simulink model "model"  (R2022a)
settings: Solver=FixedStepDiscrete  StartTime=0  StopTime=20  FixedStep=0.01  RelTol=0.00001
model workspace (MAT data in the model file):
  v0 = 0.01
undefined symbols (not defined in the file): alpha, delta, DiscIntNeverNeededParam, Fz, p, s, T, Temp, Tout, vw, ww
libraries: canmsglib x10, MoTeCM1Package x10, simulink x2, slpidlib x1
settings Model: Creator=23326  LastModifiedBy=22793
settings OptimizationCC: LifeSpan=inf
settings DebuggingCC: AlgebraicLoopMsg=none  ArtificialAlgebraicLoopMsg=none  UnconnectedInputMsg=warning  UnconnectedOutputMsg=warning  UnconnectedLineMsg=warning  SFMachineParentedDataDiag=warning  ArithmeticOperatorsInVariantConditions=warning
settings SFSimCC: CustomCodeUndefinedFunction=UseInterfaceOnly
settings CodeAppCC: StateflowObjectComments=on

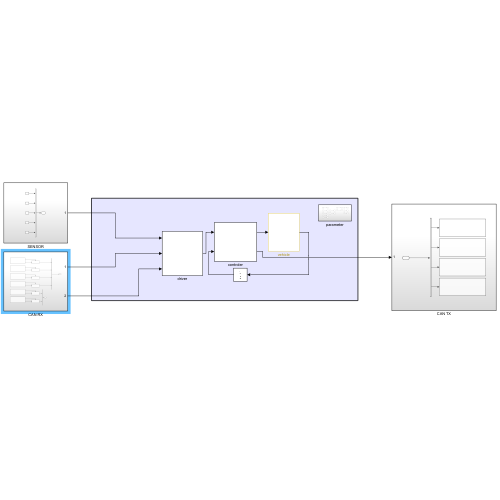
[thumbnail: Simulink's stored preview of the top-level diagram]
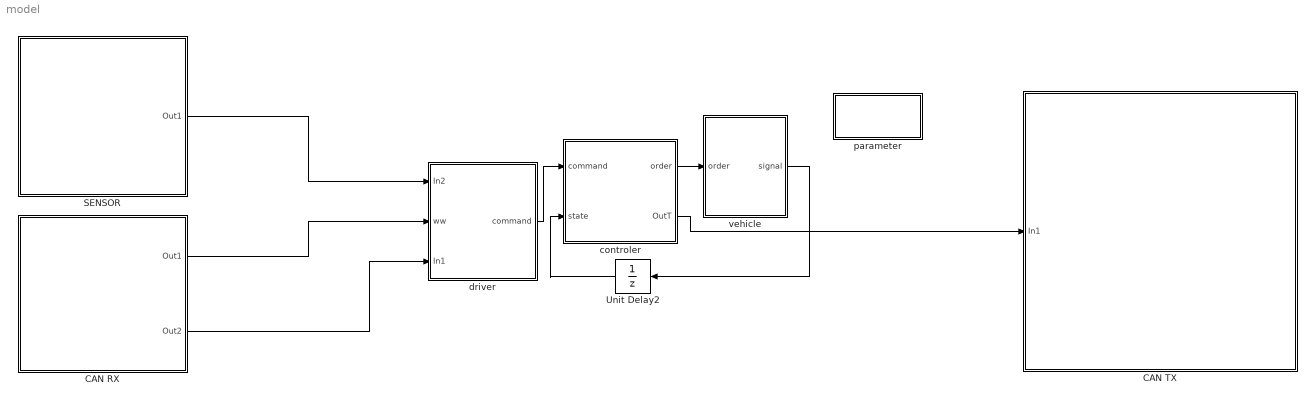
== system model ==
  CAN RX : Subsystem
  CAN TX : Subsystem
  SENSOR : Subsystem
  Unit Delay2 : UnitDelay  SampleTime=-1  HasFrameUpgradeWarning=on
  controler : Subsystem
  driver : Subsystem
  parameter : Subsystem
  vehicle : Subsystem
  wires:
  driver/1(command) -> controler/1(command)
  controler/1(order) -> vehicle/1(order)
  vehicle/1(signal) -> Unit Delay2/1
  Unit Delay2/1 -> controler/2(state)
  controler/2(OutT) -> CAN TX/1(In1)
  SENSOR/1(Out1) -> driver/1(In2)
  CAN RX/1(Out1) -> driver/2(ww)
  CAN RX/2(Out2) -> driver/3(In1)

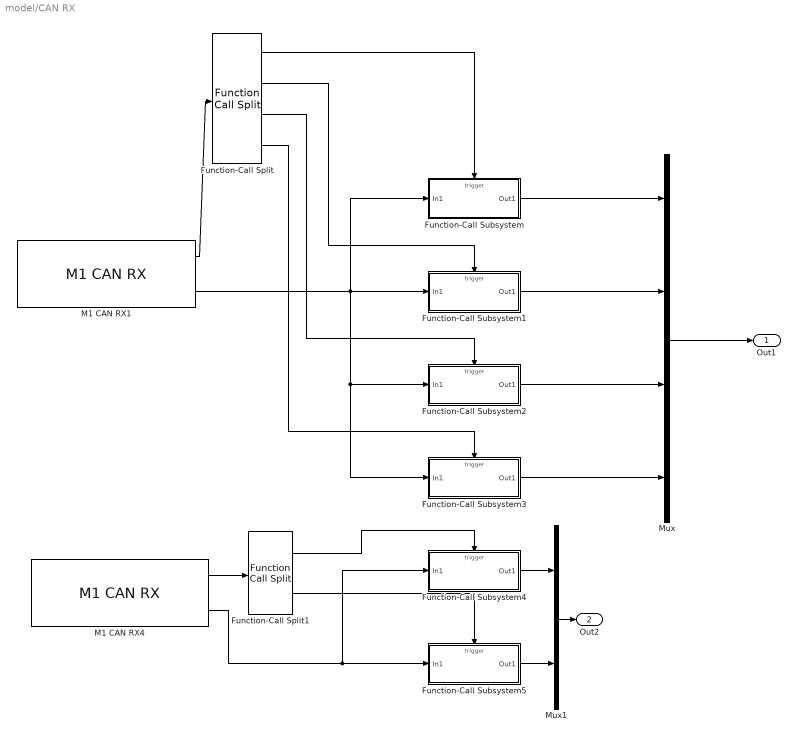
== system model/CAN RX ==
  Function-Call Split : FunctionCallSplit  IconShape=distinctive  NumOutputPorts=4  OutputPortLayout=default
  Function-Call Split1 : FunctionCallSplit  IconShape=distinctive  NumOutputPorts=2  OutputPortLayout=default
  Function-Call Subsystem : Subsystem  TreatAsAtomicUnit=on
  Function-Call Subsystem1 : Subsystem  TreatAsAtomicUnit=on
  Function-Call Subsystem2 : Subsystem  TreatAsAtomicUnit=on
  Function-Call Subsystem3 : Subsystem  TreatAsAtomicUnit=on
  Function-Call Subsystem4 : Subsystem  TreatAsAtomicUnit=on
  Function-Call Subsystem5 : Subsystem  TreatAsAtomicUnit=on
  M1 CAN RX1 : MoTeCM1Package/M1 CAN RX  CANBus=CAN Bus 1  CANFilter=Standard IDs Only  CANIDs=0  SampleTime=-1
      settings: SourceProductName=MoTeC
  M1 CAN RX4 : MoTeCM1Package/M1 CAN RX  CANBus=CAN Bus 1  CANFilter=Standard IDs Only  CANIDs=0  SampleTime=-1
      settings: SourceProductName=MoTeC
  Mux : Mux
  Mux1 : Mux  Inputs=2
  Out1 : Outport
  Out2 : Outport  Port=2
  wires:
  Function-Call Subsystem/1(Out1) -> Mux/1
  Function-Call Subsystem1/1(Out1) -> Mux/2
  Function-Call Subsystem2/1(Out1) -> Mux/3
  Function-Call Subsystem3/1(Out1) -> Mux/4
  Mux/1 -> Out1/1
  Function-Call Subsystem4/1(Out1) -> Mux1/1
  Function-Call Subsystem5/1(Out1) -> Mux1/2
  Mux1/1 -> Out2/1
  Function-Call Split/1 -> Function-Call Subsystem/Trigger
  Function-Call Split/2 -> Function-Call Subsystem1/Trigger
  Function-Call Split/3 -> Function-Call Subsystem2/Trigger
  M1 CAN RX1/2 -> Function-Call Subsystem1/1(In1), Function-Call Subsystem/1(In1), Function-Call Subsystem2/1(In1), Function-Call Subsystem3/1(In1)
  Function-Call Split/4 -> Function-Call Subsystem3/Trigger
  M1 CAN RX4/2 -> Function-Call Subsystem4/1(In1), Function-Call Subsystem5/1(In1)
  Function-Call Split1/2 -> Function-Call Subsystem5/Trigger
  M1 CAN RX1/1 -> Function-Call Split/1
  M1 CAN RX4/1 -> Function-Call Split1/1
  Function-Call Split1/1 -> Function-Call Subsystem4/Trigger

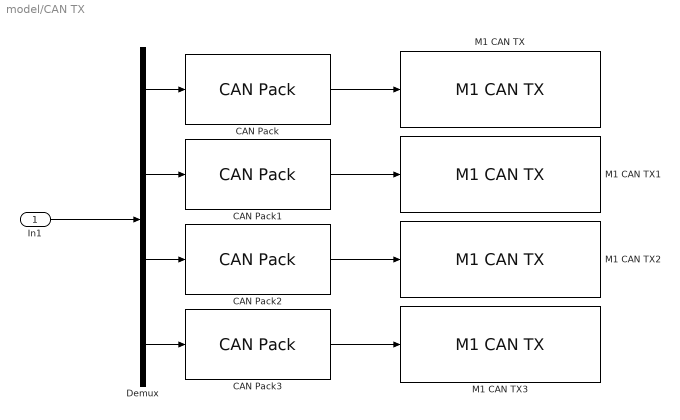
== system model/CAN TX ==
  In1 : Inport
  CAN Pack : canmsglib/CAN Pack  MsgList=(none)  MsgName=CAN Msg  MsgIDType=Standard (11-bit identifier)  MsgIdentifier=0x184  MsgLength=8  Remote=off  ApplyMinMax=off  BusOutput=off  SignalInfo={ 'Signal1', '0', '8', 'LE', 'signed', 'Standard', '0', '1', '32', '-Inf', 'Inf' }
      settings: SourceProductBaseCode=XP,ME,VN  DataFormat=manually specified signals
  CAN Pack1 : canmsglib/CAN Pack  MsgList=(none)  MsgName=CAN Msg  MsgIDType=Standard (11-bit identifier)  MsgIdentifier=0x185  MsgLength=8  Remote=off  ApplyMinMax=off  BusOutput=off  SignalInfo={ 'Signal1', '0', '8', 'LE', 'signed', 'Standard', '0', '1', '32', '-Inf', 'Inf' }
      settings: SourceProductBaseCode=XP,ME,VN  DataFormat=manually specified signals
  CAN Pack2 : canmsglib/CAN Pack  MsgList=(none)  MsgName=CAN Msg  MsgIDType=Standard (11-bit identifier)  MsgIdentifier=0x188  MsgLength=8  Remote=off  ApplyMinMax=off  BusOutput=off  SignalInfo={ 'Signal1', '0', '8', 'LE', 'signed', 'Standard', '0', '1', '32', '-Inf', 'Inf' }
      settings: SourceProductBaseCode=XP,ME,VN  DataFormat=manually specified signals
  CAN Pack3 : canmsglib/CAN Pack  MsgList=(none)  MsgName=CAN Msg  MsgIDType=Standard (11-bit identifier)  MsgIdentifier=0x189  MsgLength=8  Remote=off  ApplyMinMax=off  BusOutput=off  SignalInfo={ 'Signal1', '0', '8', 'LE', 'signed', 'Standard', '0', '1', '32', '-Inf', 'Inf' }
      settings: SourceProductBaseCode=XP,ME,VN  DataFormat=manually specified signals
  Demux : Demux
  M1 CAN TX{,1..3} (4 alike) : MoTeCM1Package/M1 CAN TX  CANBus=CAN Bus 2
      settings: SourceProductName=MoTeC
  wires:
  In1/1 -> Demux/1
  CAN Pack/1 -> M1 CAN TX/1
  Demux/1 -> CAN Pack/1
  Demux/2 -> CAN Pack1/1
  CAN Pack1/1 -> M1 CAN TX1/1
  Demux/3 -> CAN Pack2/1
  CAN Pack2/1 -> M1 CAN TX2/1
  Demux/4 -> CAN Pack3/1
  CAN Pack3/1 -> M1 CAN TX3/1

== system model/SENSOR ==
  Analogue Voltage : MoTeCM1Package/Analogue Voltage  Unit=V  DPS=3  VoltageUpdateRate=10 Hz  SensorUpdateRate=10 Hz  ValType=None  ValMinOn=on  ValMin=0  ValMaxOn=on  ValMax=0  LogRate=Default (Scheduled Rate)  DiagnosticLog=off  DiagnosticLogRate=Default (Log Rate)  SimValue=0  SimStatus=0  SimDiagnostic=0  SimVoltage=0  CRC=1061432025
      settings: SourceProductName=MoTeC
  Analogue Voltage1 : MoTeCM1Package/Analogue Voltage  Unit=V  DPS=3  VoltageUpdateRate=10 Hz  SensorUpdateRate=10 Hz  ValType=None  ValMinOn=on  ValMin=0  ValMaxOn=on  ValMax=0  LogRate=Default (Scheduled Rate)  DiagnosticLog=off  DiagnosticLogRate=Default (Log Rate)  SimValue=0  SimStatus=0  SimDiagnostic=0  SimVoltage=0  CRC=1061432025
      settings: SourceProductName=MoTeC
  Analogue Voltage2 : MoTeCM1Package/Analogue Voltage  Unit=V  DPS=3  VoltageUpdateRate=10 Hz  SensorUpdateRate=10 Hz  ValType=None  ValMinOn=on  ValMin=0  ValMaxOn=on  ValMax=0  LogRate=Default (Scheduled Rate)  DiagnosticLog=off  DiagnosticLogRate=Default (Log Rate)  SimValue=0  SimStatus=0  SimDiagnostic=0  SimVoltage=0  CRC=1061432025
      settings: SourceProductName=MoTeC
  Dual Potentiometer Pedal : MoTeCM1Package/Dual Potentiometer Pedal  Unit=ratio  DPS=3  SensorUpdateRate=50 Hz  ValType=None  ValMinOn=on  ValMin=0  ValMaxOn=on  ValMax=0  LogRate=Default (Scheduled Rate)  DiagnosticLog=off  DiagnosticLogRate=Default (Log Rate)  SimValue=0  SimStatus=0  SimDiagnostic=0  SimMainVoltage=0  SimTrackingVoltage=0  CRC=1697510422
      settings: SourceProductName=MoTeC
  Mux : Mux  Inputs=5
  Out1 : Outport
  wires:
  Analogue Voltage/1 -> Mux/3
  Mux/1 -> Out1/1
  Dual Potentiometer Pedal/1 -> Mux/2, Mux/1
  Analogue Voltage1/1 -> Mux/4
  Analogue Voltage2/1 -> Mux/5

== system model/controler ==
  command : Inport
  state : Inport  Port=2
  Bus Selector : BusSelector  OutputSignals=T
  Constant : Constant  Value=123.9
  Divide : Product  Inputs=*/
  Subsystem : Subsystem
  order : Outport
  OutT : Outport  Port=2
  wires:
  command/1 -> Subsystem/1(Command)
  state/1 -> Subsystem/2(State)
  Subsystem/1(order) -> Bus Selector/1, order/1
  Divide/1 -> OutT/1
  Bus Selector/1 -> Divide/1  "<T>"
  Constant/1 -> Divide/2

== system model/driver ==
  In2 : Inport
  ww : Inport  Port=2
  In1 : Inport  Port=3
  Bus Creator : BusCreator  Inputs=Tout,delta,Temp
  Constant2 : Constant  Value=50
  Demux : Demux  Outputs=5
  Mux : Mux  Inputs=2
  T_control : Subsystem
  command : Outport
  wires:
  Bus Creator/1 -> command/1
  Mux/1 -> Bus Creator/2  "delta"
  Constant2/1 -> Mux/2
  T_control/1(Tout) -> Bus Creator/1  "Tout"
  ww/1 -> T_control/4(ww)
  In1/1 -> Bus Creator/3
  Demux/1 -> T_control/1(Racc)
  Demux/2 -> T_control/2(Lacc)
  Demux/3 -> T_control/3(Brake)
  Demux/4 -> T_control/5(SOC)
  Demux/5 -> Mux/1
  In2/1 -> Demux/1

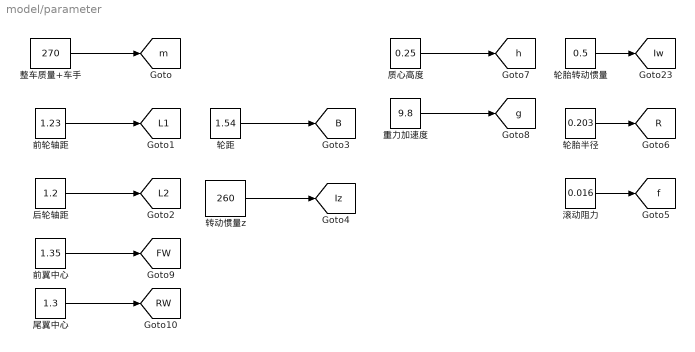
== system model/parameter ==
  前翼中心 : Constant  Value=1.35  OutDataTypeStr=double
  前轮轴距 : Constant  Value=1.23  OutDataTypeStr=double
  后轮轴距 : Constant  Value=1.2  OutDataTypeStr=double
  尾翼中心 : Constant  Value=1.3  OutDataTypeStr=double
  整车质量+车手 : Constant  Value=270  OutDataTypeStr=double
  滚动阻力 : Constant  Value=0.016  OutDataTypeStr=double
  质心高度 : Constant  Value=0.25  OutDataTypeStr=double
  转动惯量z : Constant  Value=260  OutDataTypeStr=double
  轮胎半径 : Constant  Value=0.203  OutDataTypeStr=double
  轮胎转动惯量 : Constant  Value=0.5  OutDataTypeStr=double
  轮距 : Constant  Value=1.54  OutDataTypeStr=double
  重力加速度 : Constant  Value=9.8  OutDataTypeStr=double
  tag scope: B=global, FW=global, Iw=global, Iz=global, L1=global, L2=global, R=global, RW=global, f=global, g=global, h=global, m=global
  wires:
  滚动阻力/1 -> [f]
  轮胎转动惯量/1 -> [Iw]
  整车质量+车手/1 -> [m]
  轮胎半径/1 -> [R]
  后轮轴距/1 -> [L2]
  质心高度/1 -> [h]
  转动惯量z/1 -> [Iz]
  前轮轴距/1 -> [L1]
  轮距/1 -> [B]
  重力加速度/1 -> [g]
  前翼中心/1 -> [FW]
  尾翼中心/1 -> [RW]

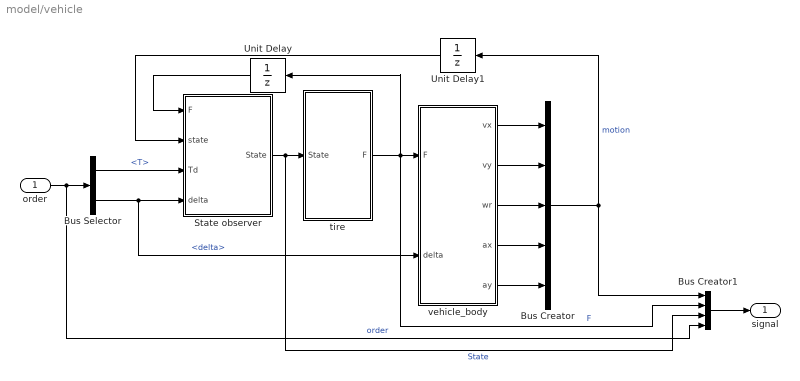
== system model/vehicle ==
  order : Inport
  Bus Creator : BusCreator  Inputs=5
  Bus Creator1 : BusCreator  Inputs=4
  Bus Selector : BusSelector  OutputSignals=T,delta
  State observer : Subsystem
  Unit Delay : UnitDelay  SampleTime=-1  HasFrameUpgradeWarning=on
  Unit Delay1 : UnitDelay  SampleTime=-1  HasFrameUpgradeWarning=on
  tire : Subsystem
  vehicle_body : Subsystem
  signal : Outport
  wires:
  vehicle_body/3(wr) -> Bus Creator/3
  vehicle_body/2(vy) -> Bus Creator/2
  tire/1(F) -> Unit Delay/1, Bus Creator1/2, vehicle_body/1(F)  "F"
  vehicle_body/4(ax) -> Bus Creator/4
  vehicle_body/5(ay) -> Bus Creator/5
  Bus Creator/1 -> Bus Creator1/1, Unit Delay1/1  "motion"
  order/1 -> Bus Creator1/4, Bus Selector/1  "order"
  Bus Selector/1 -> State observer/3(Td)  "<T>"
  Bus Selector/2 -> State observer/4(delta), vehicle_body/2(delta)  "<delta>"
  vehicle_body/1(vx) -> Bus Creator/1
  State observer/1(State) -> Bus Creator1/3, tire/1(State)  "State"
  Bus Creator1/1 -> signal/1
  Unit Delay/1 -> State observer/1(F)
  Unit Delay1/1 -> State observer/2(state)

== system model/CAN RX/Function-Call Subsystem ==
  In1 : Inport
  function : TriggerPort  TriggerType=function-call  VariantControl=(inherit)
  CAN Unpack : canmsglib/CAN Unpack  MsgList=(none)  MsgName=CAN Msg  MsgIDType=Standard (11-bit identifier)  MsgIdentifier=0x283  MsgLength=8  SignalInfo={ 'Signal1', '0', '8', 'LE', 'signed', 'Standard', '0', '1', '16', '-Inf', 'Inf' }  IDPort=off  TimestampPort=off  ErrorPort=off  RemotePort=off  LengthPort=off  StatusPort=off  ApplyMinMax=off
      settings: SourceProductBaseCode=XP,ME,VN
  Out1 : Outport
  wires:
  CAN Unpack/1 -> Out1/1
  In1/1 -> CAN Unpack/1

== system model/CAN RX/Function-Call Subsystem1 ==
  In1 : Inport
  function : TriggerPort  TriggerType=function-call  VariantControl=(inherit)
  CAN Unpack : canmsglib/CAN Unpack  MsgList=(none)  MsgName=CAN Msg  MsgIDType=Standard (11-bit identifier)  MsgIdentifier=0x284  MsgLength=8  SignalInfo={ 'Signal1', '0', '8', 'LE', 'signed', 'Standard', '0', '1', '16', '-Inf', 'Inf' }  IDPort=off  TimestampPort=off  ErrorPort=off  RemotePort=off  LengthPort=off  StatusPort=off  ApplyMinMax=off
      settings: SourceProductBaseCode=XP,ME,VN
  Out1 : Outport
  wires:
  CAN Unpack/1 -> Out1/1
  In1/1 -> CAN Unpack/1

== system model/CAN RX/Function-Call Subsystem2 ==
  In1 : Inport
  function : TriggerPort  TriggerType=function-call  VariantControl=(inherit)
  CAN Unpack : canmsglib/CAN Unpack  MsgList=(none)  MsgName=CAN Msg  MsgIDType=Standard (11-bit identifier)  MsgIdentifier=0x287  MsgLength=8  SignalInfo={ 'Signal1', '0', '8', 'LE', 'signed', 'Standard', '0', '1', '16', '-Inf', 'Inf' }  IDPort=off  TimestampPort=off  ErrorPort=off  RemotePort=off  LengthPort=off  StatusPort=off  ApplyMinMax=off
      settings: SourceProductBaseCode=XP,ME,VN
  Out1 : Outport
  wires:
  In1/1 -> CAN Unpack/1
  CAN Unpack/1 -> Out1/1

== system model/CAN RX/Function-Call Subsystem3 ==
  In1 : Inport
  function : TriggerPort  TriggerType=function-call  VariantControl=(inherit)
  CAN Unpack : canmsglib/CAN Unpack  MsgList=(none)  MsgName=CAN Msg  MsgIDType=Standard (11-bit identifier)  MsgIdentifier=0x288  MsgLength=8  SignalInfo={ 'Signal1', '0', '8', 'LE', 'signed', 'Standard', '0', '1', '16', '-Inf', 'Inf' }  IDPort=off  TimestampPort=off  ErrorPort=off  RemotePort=off  LengthPort=off  StatusPort=off  ApplyMinMax=off
      settings: SourceProductBaseCode=XP,ME,VN
  Out1 : Outport
  wires:
  In1/1 -> CAN Unpack/1
  CAN Unpack/1 -> Out1/1

== system model/CAN RX/Function-Call Subsystem4 ==
  In1 : Inport
  function : TriggerPort  TriggerType=function-call  VariantControl=(inherit)
  CAN Unpack : canmsglib/CAN Unpack  MsgList=(none)  MsgName=CAN Msg  MsgIDType=Standard (11-bit identifier)  MsgIdentifier=0x289  MsgLength=8  SignalInfo={ 'Signal1', '0', '8', 'LE', 'signed', 'Standard', '0', '1', '16', '-Inf', 'Inf' }  IDPort=off  TimestampPort=off  ErrorPort=off  RemotePort=off  LengthPort=off  StatusPort=off  ApplyMinMax=off
      settings: SourceProductBaseCode=XP,ME,VN
  Out1 : Outport
  wires:
  In1/1 -> CAN Unpack/1
  CAN Unpack/1 -> Out1/1

== system model/CAN RX/Function-Call Subsystem5 ==
  In1 : Inport
  function : TriggerPort  TriggerType=function-call  VariantControl=(inherit)
  CAN Unpack : canmsglib/CAN Unpack  MsgList=(none)  MsgName=CAN Msg  MsgIDType=Standard (11-bit identifier)  MsgIdentifier=0x290  MsgLength=8  SignalInfo={ 'Signal1', '0', '8', 'LE', 'signed', 'Standard', '0', '1', '16', '-Inf', 'Inf' }  IDPort=off  TimestampPort=off  ErrorPort=off  RemotePort=off  LengthPort=off  StatusPort=off  ApplyMinMax=off
      settings: SourceProductBaseCode=XP,ME,VN
  Out1 : Outport
  wires:
  In1/1 -> CAN Unpack/1
  CAN Unpack/1 -> Out1/1

== system model/controler/Subsystem ==
  Command : Inport
  State : Inport  Port=2
  Bus Creator : BusCreator  Inputs=delta,T,p
  Bus Selector : BusSelector  OutputSignals=Tout,delta,Temp
  Bus Selector1 : BusSelector  OutputSignals=State.Fz,State.ww,motion.vx,motion.wr
  Demux : Demux  Outputs=2
  MATLAB Function : MATLAB Function  TreatAsAtomicUnit=on
  Mux : Mux  Inputs=2
  Subsystem : Subsystem
  order : Outport
  wires:
  State/1 -> Bus Selector1/1
  Bus Selector1/1 -> Subsystem/2(Fz)  "<Fz>"
  Bus Selector/1 -> Subsystem/1(Req_T)  "<Tout>"
  Command/1 -> Bus Selector/1
  Bus Selector/2 -> Demux/1, Subsystem/4(delta)  "<delta>"
  Subsystem/2(p) -> Bus Creator/3
  Bus Creator/1 -> order/1
  Subsystem/1(T) -> Bus Creator/2  "T"
  Demux/1 -> MATLAB Function/1(u1)
  Demux/2 -> MATLAB Function/2(u2)
  MATLAB Function/1(f) -> Mux/1
  MATLAB Function/2(r) -> Mux/2
  Mux/1 -> Bus Creator/1  "delta"
  Bus Selector/3 -> Subsystem/3(Temp)  "<Temp>"
  Bus Selector1/2 -> Subsystem/5(ww)  "<ww>"
  Bus Selector1/4 -> Subsystem/7(wreal)  "<wr>"
  Bus Selector1/3 -> Subsystem/6(vx)  "<vx>"

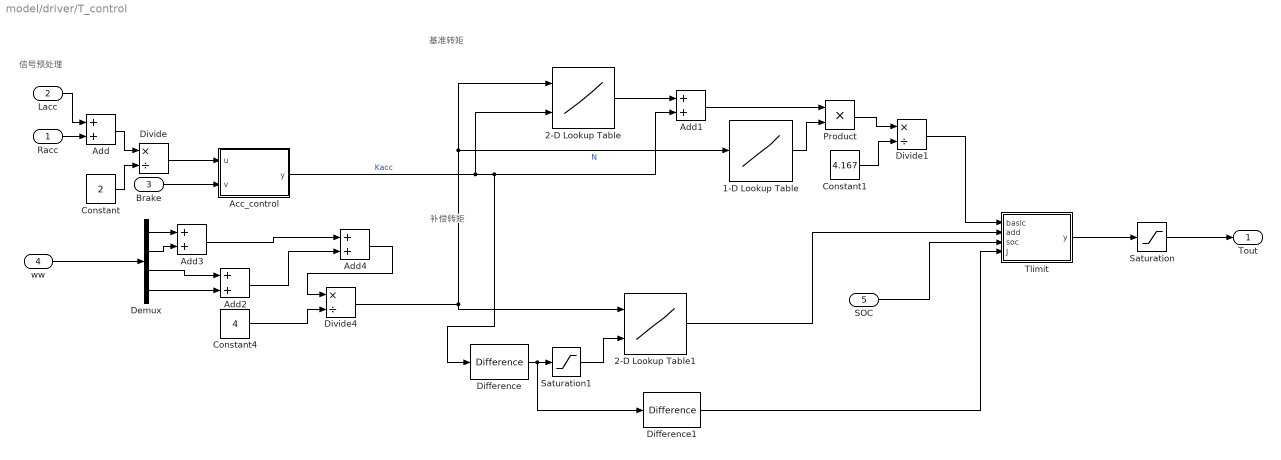
== system model/driver/T_control ==
  note: 补偿转矩
  note: 信号预处理
  note: 基准转矩
  Racc : Inport  OutDataTypeStr=double
  Lacc : Inport  Port=2  OutDataTypeStr=double
  Brake : Inport  Port=3
  ww : Inport  Port=4
  SOC : Inport  Port=5
  1-D Lookup Table : Lookup_n-D  NumberOfTableDimensions=1  BreakpointsForDimension1=[0;1000;2000;3000;4000;5000;6000;7000;8000;9000;10000;11000;12000;13000;14000;15000;16000;17000;18000;19000]  Table=[21;21;21;21;21;21;21;21;21;21;21;21;21;21;20;18;15;13;9.8;0]  InternalRulePriority=Speed  RndMeth=Simplest
  2-D Lookup Table : Lookup_n-D  BreakpointsForDimension1=[0 1000 2000 3000 4000 5000 6000 7000 8000 9000 10000 12000 14000]  BreakpointsForDimension2=[0 5 10 20 30 40 50 60 70 80 90 95 100]  BreakpointsForDimension1FirstPoint=0  BreakpointsForDimension2FirstPoint=0  BreakpointsForDimension1Spacing=1000  BreakpointsForDimension2Spacing=10  Table=[0.315789474 0.653846154 0.703703704 0.80952381 1.052631579 1.194444444 1.302083333 1.507246377 1.564102564 1.507246377 1.564102564 1.527777778 1.564102564;0.342857143 0.666666667 0.666666667 0.768707483 0.930232558 1.068181818 1.088888889 1.419354839 1.419354839 1.419354839 1.419354839 1.419354839 1.507246377;0.315789474 0.513888889 0.533333333 0.62601626 0.583333333 0.422222222 0.627118644 0.871794872 1.052631579 1.147058824 1.225 1.236842105 1.302083333;0.150537634 0.333333333 0.333333333 0.333333333 0.263565891 0.031446541 0.333333333 0.698113208 0.930232558 1.023809524 1.088888889 1.088888889 1.216216216;0.137254902 0.257575758 0.173333333 0.141843972 -0.083333333 -0.31372549 -0.133333333 0.122807018 0.346666667 0.468085106 0.589285714 0.847826087 1.138888889;0.150537634 0.263565891 0.141843972 1.34572e-17 -0.210884354 -0.635220126 -0.542372881 -0.303030303 6.72862e-17 0.237288136 0.58490566 0.837037037 1.121212121;0.137254902 0.12962963 5.28678e-17 -0.141843972 -0.310606061 -0.777777778 -0.724637681 -0.549019608 -0.217391304 0.237288136 0.589285714 0.847826087 1.138888889;1.37065e-17 -0.08045977 -0.212121212 -0.333333333 -0.403100775 -0.635220126 -0.866666667 -0.974358974 -0.290598291 0.237288136 0.58490566 0.837037037 1;1.23358e-17 -0.077777778 -0.194444444 -0.212121212 -0.280701754 -0.511111111 -0.69005848 -0.549019608 -0.217391304 0.192982456 0.4375 0.692982456 0.861111111;1.37065e-17 -0.08045977 -0.212121212 -0.333333333 -0.333333333 -0.333333333 -0.542372881 -0.303030303 -0.06918239 1.45127e-17 0.205128205 0.47311828 0.666666667;-0.194444444 -0.205882353 -0.194444444 -0.333333333 -0.472222222 -0.454545455 -0.385964912 -0.078431373 0.143939394 0.205128205 0.238095238 0.37037037 0.472222222;-0.333333333 -0.333333333 -0.333333333 -0.333333333 -0.454545455 -0.358974359 -0.2 0.333333333 0.333333333 0.333333333 0.333333333 0.333333333 0.333333333;-0.472222222 -0.460784314 -0.472222222 -0.454545455 -0.472222222 -0.358974359 -0.058333333 0.212121212 0.194444444 0.212121212 0.194444444 0.205882353 0.194444444]  InternalRulePriority=Speed  RndMeth=Simplest
      settings: InputPortMap=u0,u1
  2-D Lookup Table1 : Lookup_n-D  BreakpointsForDimension1=[0;1000;2000;3000;4000;5000;6000;7000;8000;9000;10000;11000;12000;13000;14000]  BreakpointsForDimension2=[-50;-25;0;25;50]  Table=[0 0 0 4 5;0 0 0 4 5;0 0 0 4 5;0 0 0 4 5;-3 -2 0 4 5;-3 -2 0 3 5;-3 -2 0 3 4;-3 -2 0 3 4;-4 -3 0 2 3;-4 -3 0 2 3;-5 -3 0 1 2;-5 -4 0 1 2;-5 -4 0 0 0;-5 -4 0 0 0;-5 -4 0 0 0]  InternalRulePriority=Speed  RndMeth=Simplest
      settings: InputPortMap=u0,u1
  Acc_control : MATLAB Function  TreatAsAtomicUnit=on
  Add{,1..4} (5 alike) : Sum
  Constant : Constant  Value=2  OutDataTypeStr=uint8
  Constant1 : Constant  Value=4.167
  Constant4 : Constant  Value=4
  Demux : Demux
  Difference : simulink/Discrete/Difference  ICPrevInput=0.0  OutMin=[]  OutMax=[]  OutDataType=fixdt(1, 16)  OutScaling=2^-10  DoSatur=off
  Difference1 : simulink/Discrete/Difference  ICPrevInput=0.0  OutMin=[]  OutMax=[]  OutDataType=fixdt(1, 16)  OutScaling=2^-10  DoSatur=off
  Divide : Product  Inputs=*/
  Divide1 : Product  Inputs=*/
  Divide4 : Product  Inputs=*/
  Product : Product
  Saturation : Saturate  UpperLimit=495  LowerLimit=0
  Saturation1 : Saturate  UpperLimit=50  LowerLimit=-50
  Tlimit : MATLAB Function  TreatAsAtomicUnit=on
  Tout : Outport
  wires:
  Lacc/1 -> Add/1
  Racc/1 -> Add/2
  Add/1 -> Divide/1
  Constant/1 -> Divide/2
  Brake/1 -> Acc_control/2(v)
  Divide/1 -> Acc_control/1(u)
  SOC/1 -> Tlimit/3(soc)
  Difference/1 -> Difference1/1, Saturation1/1
  Difference1/1 -> Tlimit/4(J)
  1-D Lookup Table/1 -> Product/2
  2-D Lookup Table/1 -> Add1/1
  Demux/3 -> Add2/1
  Demux/4 -> Add2/2
  Constant4/1 -> Divide4/2
  Divide4/1 -> 2-D Lookup Table/1, 1-D Lookup Table/1, 2-D Lookup Table1/1  "N"
  Acc_control/1(y) -> 2-D Lookup Table/2, Difference/1, Add1/2  "Kacc"
  Demux/1 -> Add3/1
  Demux/2 -> Add3/2
  Add3/1 -> Add4/1
  Add2/1 -> Add4/2
  Add4/1 -> Divide4/1
  Saturation/1 -> Tout/1
  Tlimit/1(y) -> Saturation/1
  Saturation1/1 -> 2-D Lookup Table1/2
  Add1/1 -> Product/1
  Product/1 -> Divide1/1
  Constant1/1 -> Divide1/2
  Divide1/1 -> Tlimit/1(basic)
  ww/1 -> Demux/1
  2-D Lookup Table1/1 -> Tlimit/2(add)

== system model/vehicle/State observer ==
  F : Inport
  state : Inport  Port=2
  Td : Inport  Port=3
  delta : Inport  Port=4
  Bus Creator : BusCreator  Inputs=alpha,s,Fz,ww,vw
  Fz : Subsystem
  alpha&vw : Subsystem
  lamda : Subsystem
  wheel : Subsystem
  State : Outport
  wires:
  alpha&vw/1(alpha) -> Bus Creator/1  "alpha"
  Fz/1(Fz) -> wheel/3(Fz), Bus Creator/3  "Fz"
  alpha&vw/2(vw) -> Bus Creator/5, lamda/1(vw)  "vw"
  wheel/1(ww) -> lamda/2(ww), Bus Creator/4  "ww"
  lamda/1(s) -> Bus Creator/2  "s"
  state/1 -> alpha&vw/2(state), Fz/1(state)
  Td/1 -> wheel/1(Td)  "Td"
  Bus Creator/1 -> State/1
  F/1 -> wheel/2(F)
  delta/1 -> alpha&vw/1(delta)

== system model/vehicle/tire ==
  State : Inport
  Bus Creator : BusCreator  Inputs=8
  Bus Selector : BusSelector  OutputSignals=alpha,s,Fz
  MATLAB Function3 : MATLAB Function  TreatAsAtomicUnit=on
  F : Outport
  wires:
  MATLAB Function3/1(Fx1) -> Bus Creator/1
  MATLAB Function3/4(Fx4) -> Bus Creator/4
  MATLAB Function3/3(Fx3) -> Bus Creator/3
  MATLAB Function3/2(Fx2) -> Bus Creator/2
  MATLAB Function3/5(Fy1) -> Bus Creator/5
  MATLAB Function3/6(Fy2) -> Bus Creator/6
  MATLAB Function3/7(Fy3) -> Bus Creator/7
  MATLAB Function3/8(Fy4) -> Bus Creator/8
  State/1 -> Bus Selector/1
  Bus Selector/1 -> MATLAB Function3/1(alpha)  "<alpha>"
  Bus Selector/2 -> MATLAB Function3/2(s)  "<s>"
  Bus Selector/3 -> MATLAB Function3/3(Fz)  "<Fz>"
  Bus Creator/1 -> F/1

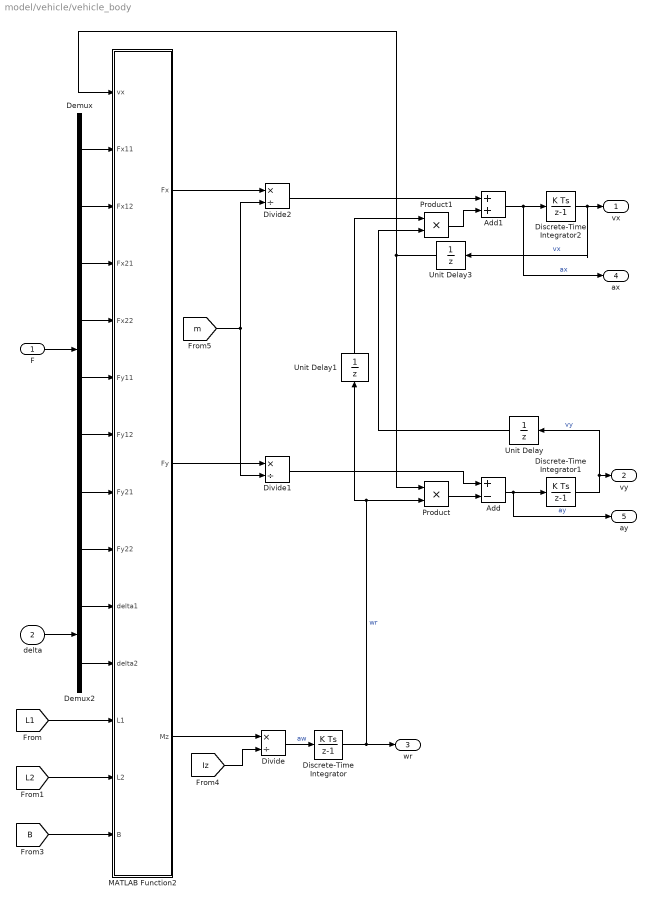
== system model/vehicle/vehicle_body ==
  F : Inport
  delta : Inport  Port=2
  Add : Sum  Inputs=+-
  Add1 : Sum
  Demux : Demux  Outputs=8
  Demux2 : Demux  Outputs=2
  Discrete-Time Integrator : DiscreteIntegrator  SampleTime=-1  ICPrevOutput=DiscIntNeverNeededParam  ICPrevScaledInput=DiscIntNeverNeededParam
  Discrete-Time Integrator1 : DiscreteIntegrator  SampleTime=-1  ICPrevOutput=DiscIntNeverNeededParam  ICPrevScaledInput=DiscIntNeverNeededParam
  Discrete-Time Integrator2 : DiscreteIntegrator  SampleTime=-1  ICPrevOutput=DiscIntNeverNeededParam  ICPrevScaledInput=DiscIntNeverNeededParam
  Divide : Product  Inputs=*/
  Divide1 : Product  Inputs=*/
  Divide2 : Product  Inputs=*/
  MATLAB Function2 : MATLAB Function  TreatAsAtomicUnit=on
  Product : Product
  Product1 : Product
  Unit Delay : UnitDelay  SampleTime=-1  HasFrameUpgradeWarning=on
  Unit Delay1 : UnitDelay  SampleTime=-1  HasFrameUpgradeWarning=on
  Unit Delay3 : UnitDelay  SampleTime=-1  HasFrameUpgradeWarning=on
  vx : Outport
  vy : Outport  Port=2
  wr : Outport  Port=3
  ax : Outport  Port=4
  ay : Outport  Port=5
  wires:
  Discrete-Time Integrator1/1 -> Unit Delay/1, vy/1  "vy"
  Discrete-Time Integrator/1 -> Product/2, Unit Delay1/1, wr/1  "wr"
  Divide/1 -> Discrete-Time Integrator/1  "aw"
  Discrete-Time Integrator2/1 -> vx/1, Unit Delay3/1  "vx"
  Demux2/2 -> MATLAB Function2/11(delta2)
  MATLAB Function2/3(Mz) -> Divide/1
  Add/1 -> Discrete-Time Integrator1/1, ay/1  "ay"
  Divide2/1 -> Add1/1
  Add1/1 -> Discrete-Time Integrator2/1, ax/1  "ax"
  MATLAB Function2/1(Fx) -> Divide2/1
  Divide1/1 -> Add/1
  Product1/1 -> Add1/2
  MATLAB Function2/2(Fy) -> Divide1/1
  Product/1 -> Add/2
  delta/1 -> Demux2/1
  F/1 -> Demux/1
  Demux2/1 -> MATLAB Function2/10(delta1)
  [L1] -> MATLAB Function2/12(L1)
  [L2] -> MATLAB Function2/13(L2)
  [B] -> MATLAB Function2/14(B)
  [Iz] -> Divide/2
  [m] -> Divide2/2, Divide1/2
  Demux/8 -> MATLAB Function2/9(Fy22)
  Demux/7 -> MATLAB Function2/8(Fy21)
  Demux/6 -> MATLAB Function2/7(Fy12)
  Demux/5 -> MATLAB Function2/6(Fy11)
  Demux/4 -> MATLAB Function2/5(Fx22)
  Demux/3 -> MATLAB Function2/4(Fx21)
  Demux/2 -> MATLAB Function2/3(Fx12)
  Demux/1 -> MATLAB Function2/2(Fx11)
  Unit Delay/1 -> Product1/2
  Unit Delay1/1 -> Product1/1
  Unit Delay3/1 -> MATLAB Function2/1(vx), Product/1

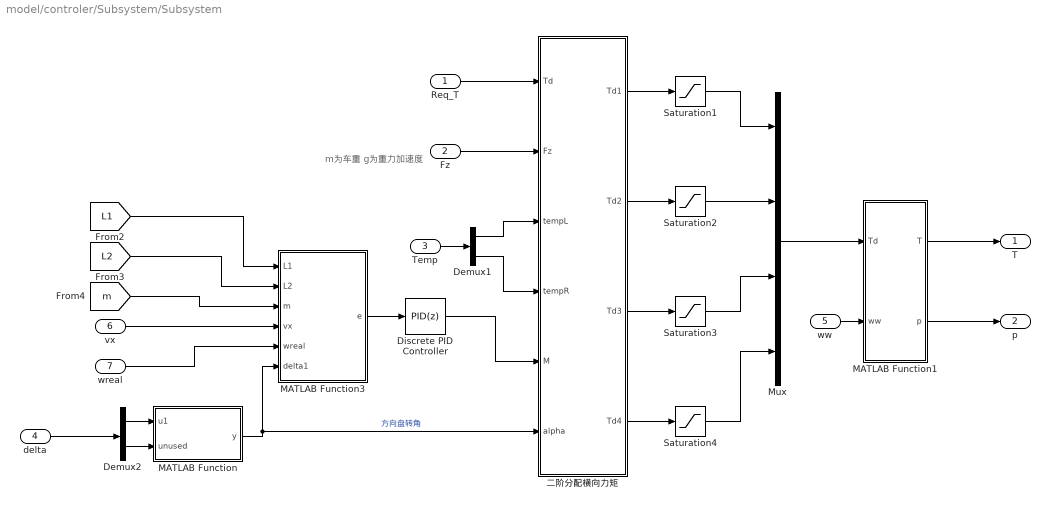
== system model/controler/Subsystem/Subsystem ==
  note: m为车重
      | g为重力加速度
  Req_T : Inport
  Fz : Inport  Port=2
  Temp : Inport  Port=3
  delta : Inport  Port=4
  ww : Inport  Port=5
  vx : Inport  Port=6
  wreal : Inport  Port=7
  Demux1 : Demux  Outputs=2
  Demux2 : Demux  Outputs=2
  Discrete PID Controller : slpidlib/PID Controller  Controller=PID  Form=Parallel  TimeDomain=Discrete-time  UseExternalTs=off  SampleTime=-1  IntegratorMethod=Forward Euler  FilterMethod=Forward Euler  ControllerParametersSource=internal  P=20  I=5  UseKiTs=off  D=2  N=20  UseFilter=on  TunerSelectOption=Frequency Response Based  InitialConditionSource=internal  InitialConditionForIntegrator=0  InitialConditionForFilter=0  DifferentiatorICPrevScaledInput=0  ExternalReset=none  TrackingMode=off  Kt=1  LimitOutput=off  SatLimitsSource=internal  UpperSaturationLimit=inf  LowerSaturationLimit=-inf  LinearizeAsGain=off  AntiWindupMode=none  Kb=1  POutMin=[]  POutMax=[]  IOutMin=[]  IOutMax=[]  DOutMin=[]  DOutMax=[]  NOutMin=[]  NOutMax=[]  SumOutMin=[]  SumOutMax=[]  SaturationOutMin=[]  SaturationOutMax=[]  PParamMin=[]  PParamMax=[]  IParamMin=[]  IParamMax=[]  DParamMin=[]  DParamMax=[]  NParamMin=[]  NParamMax=[]  KbParamMin=[]  KbParamMax=[]  KtParamMin=[]  KtParamMax=[]  KbOutMin=[]  KbOutMax=[]  KtOutMin=[]  KtOutMax=[]  IntegratorOutMin=[]  IntegratorOutMax=[]  FilterOutMin=[]  FilterOutMax=[]  SumI1OutMin=[]  SumI1OutMax=[]  SumI2OutMin=[]  SumI2OutMax=[]  SumI3OutMin=[]  SumI3OutMax=[]  SumI4OutMin=[]  SumI4OutMax=[]  SumDOutMin=[]  SumDOutMax=[]  DifferentiatorOutMin=[]  DifferentiatorOutMax=[]  FilterDiffOutCoefMin=[]  FilterDiffOutCoefMax=[]  ReciprocalOutMin=[]  ReciprocalOutMax=[]  SumDenOutMin=[]  SumDenOutMax=[]  SumNumOutMin=[]  SumNumOutMax=[]  DivideOutMin=[]  DivideOutMax=[]  UdiffTsProdOutMin=[]  UdiffTsProdOutMax=[]  NTsProdOutMin=[]  NTsProdOutMax=[]  UintegralTsProdOutMin=[]  UintegralTsProdOutMax=[]  UngainTsProdOutMin=[]  UngainTsProdOutMax=[]  ClampingZeroOutDataTypeStr=Inherit: Inherit via back propagation  ClampingZeroOutMin=[]  ClampingZeroOutMax=[]  FilterDenConstantOutDataTypeStr=Inherit: Inherit via back propagation  FilterDenConstantOutMin=[]  FilterDenConstantOutMax=[]  PCopyOutDataTypeStr=Inherit: Inherit via back propagation  PCopyOutMin=[]  PCopyOutMax=[]  NCopyOutDataTypeStr=Inherit: Inherit via back propagation  NCopyOutMin=[]  NCopyOutMax=[]  IntegratorContinuousStateAttributes=''  IntegratorStateMustResolveToSignalObject=off  IntegratorRTWStateStorageClass=Auto  FilterContinuousStateAttributes=''  FilterStateMustResolveToSignalObject=off  FilterRTWStateStorageClass=Auto  ParallelPVariant=InternalParameters  IdealPVariant=Disabled  IVariant=InternalParameters  DVariant=InternalParameters  IntegratorVariant=Discrete  SatVariant=Disabled  AWVariant=Passthrough  PCopyVariant=Disabled  TRVariant=Disabled  FdbkBlocksVariant=Forward  IdealPFdbkVariant=Disabled  SatFdbkVariant=Disabled  DerivativeFilterVariant=ForwardEulerFilter  NVariant=InternalParameters  NCopyVariant=Disabled  FilterICVariant=InternalICsFilter  IntegratorICVariant=InternalICs  ExternalResetVariant=Disabled  TRSumVariant=Passthrough  SumFdbkVariant=Disabled  SumVariant=Sum_PID  TsampFilterVariant=InternalTs  TsampNgainVariant=Passthrough  TsampIntegralVariant=Passthrough  ExternalSaturationOutDataTypeStr=Inherit: Same as second input  aMode=0
  MATLAB Function : MATLAB Function  TreatAsAtomicUnit=on
  MATLAB Function1 : MATLAB Function  TreatAsAtomicUnit=on
  MATLAB Function3 : MATLAB Function  TreatAsAtomicUnit=on
  Mux : Mux
  Saturation{1..4} (4 alike) : Saturate  UpperLimit=123.9  LowerLimit=0
  二阶分配横向力矩 : MATLAB Function  TreatAsAtomicUnit=on
  T : Outport
  p : Outport  Port=2
  wires:
  Fz/1 -> 二阶分配横向力矩/2(Fz)
  Demux1/1 -> 二阶分配横向力矩/3(tempL)
  Demux2/1 -> MATLAB Function/1(u1)
  Req_T/1 -> 二阶分配横向力矩/1(Td)
  Demux1/2 -> 二阶分配横向力矩/4(tempR)
  delta/1 -> Demux2/1
  Temp/1 -> Demux1/1
  Demux2/2 -> MATLAB Function/2(unused)
  二阶分配横向力矩/1(Td1) -> Saturation1/1
  二阶分配横向力矩/2(Td2) -> Saturation2/1
  二阶分配横向力矩/3(Td3) -> Saturation3/1
  二阶分配横向力矩/4(Td4) -> Saturation4/1
  ww/1 -> MATLAB Function1/2(ww)
  Saturation1/1 -> Mux/1
  Saturation2/1 -> Mux/2
  Saturation3/1 -> Mux/3
  Saturation4/1 -> Mux/4
  Mux/1 -> MATLAB Function1/1(Td)
  MATLAB Function1/2(p) -> p/1
  MATLAB Function1/1(T) -> T/1
  vx/1 -> MATLAB Function3/4(vx)
  wreal/1 -> MATLAB Function3/5(wreal)
  [m] -> MATLAB Function3/3(m)
  [L2] -> MATLAB Function3/2(L2)
  [L1] -> MATLAB Function3/1(L1)
  MATLAB Function/1(y) -> 二阶分配横向力矩/6(alpha), MATLAB Function3/6(delta1)  "方向盘转角"
  MATLAB Function3/1(e) -> Discrete PID Controller/1
  Discrete PID Controller/1 -> 二阶分配横向力矩/5(M)

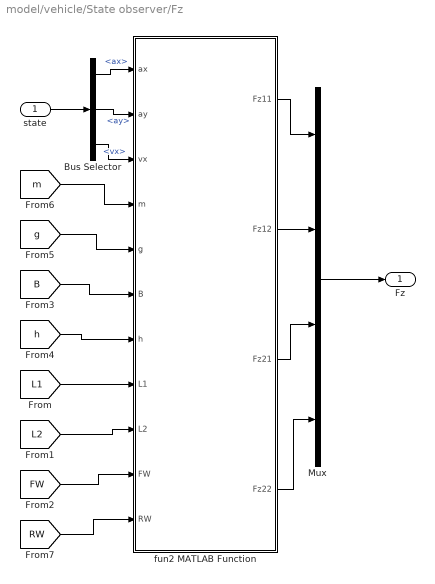
== system model/vehicle/State observer/Fz ==
  state : Inport
  Bus Selector : BusSelector  OutputSignals=ax,ay,vx
  Mux : Mux
  fun2 MATLAB Function : MATLAB Function  TreatAsAtomicUnit=on
  Fz : Outport
  wires:
  [L2] -> fun2 MATLAB Function/9(L2)
  [L1] -> fun2 MATLAB Function/8(L1)
  [h] -> fun2 MATLAB Function/7(h)
  [g] -> fun2 MATLAB Function/5(g)
  [m] -> fun2 MATLAB Function/4(m)
  Mux/1 -> Fz/1
  fun2 MATLAB Function/1(Fz11) -> Mux/1
  fun2 MATLAB Function/2(Fz12) -> Mux/2
  fun2 MATLAB Function/3(Fz21) -> Mux/3
  fun2 MATLAB Function/4(Fz22) -> Mux/4
  [B] -> fun2 MATLAB Function/6(B)
  state/1 -> Bus Selector/1
  Bus Selector/1 -> fun2 MATLAB Function/1(ax)  "<ax>"
  Bus Selector/2 -> fun2 MATLAB Function/2(ay)  "<ay>"
  Bus Selector/3 -> fun2 MATLAB Function/3(vx)  "<vx>"
  [FW] -> fun2 MATLAB Function/10(FW)
  [RW] -> fun2 MATLAB Function/11(RW)

== system model/vehicle/State observer/alpha&vw ==
  delta : Inport
  state : Inport  Port=2
  Bus Selector : BusSelector  OutputSignals=vx,vy,wr
  cepianjiao : Subsystem
  lunsu : Subsystem
  alpha : Outport
  vw : Outport  Port=2
  wires:
  lunsu/1(vw) -> vw/1
  Bus Selector/2 -> lunsu/3(vy), cepianjiao/3(vy)  "<vy>"
  cepianjiao/1(alpha) -> alpha/1
  delta/1 -> lunsu/1(delta), cepianjiao/1(delta)
  Bus Selector/1 -> cepianjiao/2(vx), lunsu/2(vx)  "<vx>"
  state/1 -> Bus Selector/1
  Bus Selector/3 -> lunsu/4(wr), cepianjiao/4(wr)  "<wr>"

== system model/vehicle/State observer/lamda ==
  vw : Inport
  ww : Inport  Port=2
  MATLAB Function2 : MATLAB Function  TreatAsAtomicUnit=on
  Mux : Mux
  s : Outport
  wires:
  [R] -> MATLAB Function2/3(R)
  vw/1 -> MATLAB Function2/1(vw)
  ww/1 -> MATLAB Function2/2(ww)
  MATLAB Function2/1(s1) -> Mux/1
  MATLAB Function2/4(s4) -> Mux/4
  MATLAB Function2/2(s2) -> Mux/2
  MATLAB Function2/3(s3) -> Mux/3
  Mux/1 -> s/1

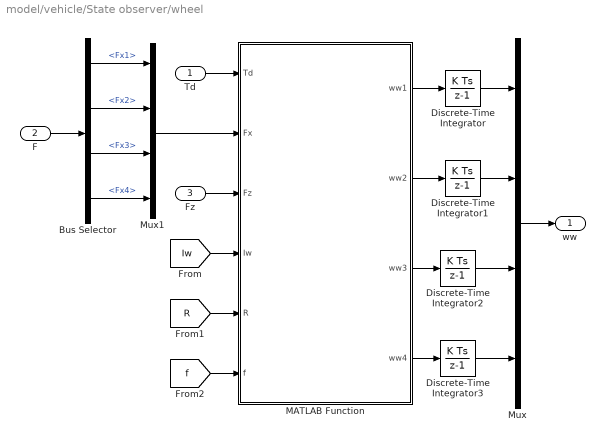
== system model/vehicle/State observer/wheel ==
  Td : Inport
  F : Inport  Port=2
  Fz : Inport  Port=3
  Bus Selector : BusSelector  OutputSignals=Fx1,Fx2,Fx3,Fx4
  Discrete-Time Integrator{,1..3} (4 alike) : DiscreteIntegrator  SampleTime=-1  ICPrevOutput=DiscIntNeverNeededParam  ICPrevScaledInput=DiscIntNeverNeededParam
  MATLAB Function : MATLAB Function  TreatAsAtomicUnit=on
  Mux : Mux
  Mux1 : Mux
  ww : Outport
  wires:
  MATLAB Function/1(ww1) -> Discrete-Time Integrator/1
  Discrete-Time Integrator/1 -> Mux/1
  Td/1 -> MATLAB Function/1(Td)
  Fz/1 -> MATLAB Function/3(Fz)
  Discrete-Time Integrator1/1 -> Mux/2
  Discrete-Time Integrator2/1 -> Mux/3
  Discrete-Time Integrator3/1 -> Mux/4
  [Iw] -> MATLAB Function/4(Iw)
  [R] -> MATLAB Function/5(R)
  [f] -> MATLAB Function/6(f)
  Mux/1 -> ww/1
  MATLAB Function/2(ww2) -> Discrete-Time Integrator1/1
  MATLAB Function/3(ww3) -> Discrete-Time Integrator2/1
  MATLAB Function/4(ww4) -> Discrete-Time Integrator3/1
  F/1 -> Bus Selector/1
  Bus Selector/1 -> Mux1/1  "<Fx1>"
  Bus Selector/2 -> Mux1/2  "<Fx2>"
  Bus Selector/3 -> Mux1/3  "<Fx3>"
  Bus Selector/4 -> Mux1/4  "<Fx4>"
  Mux1/1 -> MATLAB Function/2(Fx)

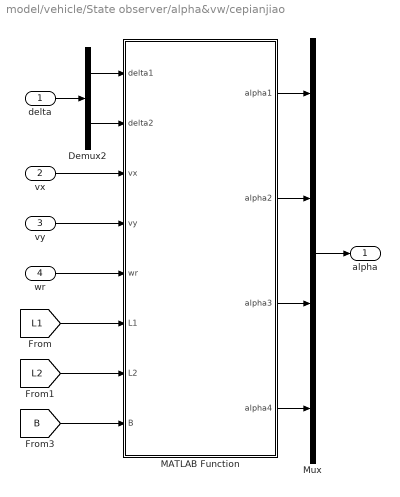
== system model/vehicle/State observer/alpha&vw/cepianjiao ==
  delta : Inport
  vx : Inport  Port=2
  vy : Inport  Port=3
  wr : Inport  Port=4
  Demux2 : Demux  Outputs=2
  MATLAB Function : MATLAB Function  TreatAsAtomicUnit=on
  Mux : Mux
  alpha : Outport
  wires:
  vy/1 -> MATLAB Function/4(vy)
  vx/1 -> MATLAB Function/3(vx)
  wr/1 -> MATLAB Function/5(wr)
  Demux2/1 -> MATLAB Function/1(delta1)
  delta/1 -> Demux2/1
  Demux2/2 -> MATLAB Function/2(delta2)
  [L1] -> MATLAB Function/6(L1)
  [L2] -> MATLAB Function/7(L2)
  [B] -> MATLAB Function/8(B)
  Mux/1 -> alpha/1
  MATLAB Function/1(alpha1) -> Mux/1
  MATLAB Function/2(alpha2) -> Mux/2
  MATLAB Function/3(alpha3) -> Mux/3
  MATLAB Function/4(alpha4) -> Mux/4

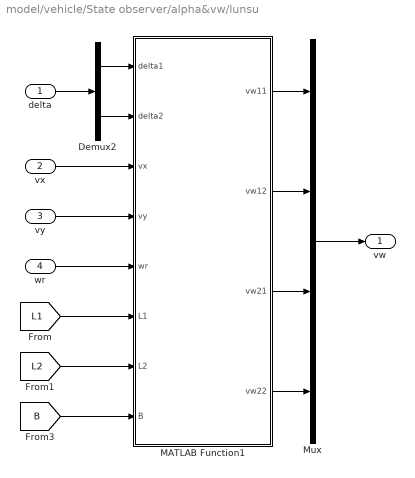
== system model/vehicle/State observer/alpha&vw/lunsu ==
  delta : Inport
  vx : Inport  Port=2
  vy : Inport  Port=3
  wr : Inport  Port=4
  Demux2 : Demux  Outputs=2
  MATLAB Function1 : MATLAB Function  TreatAsAtomicUnit=on
  Mux : Mux
  vw : Outport
  wires:
  Demux2/1 -> MATLAB Function1/1(delta1)
  vy/1 -> MATLAB Function1/4(vy)
  vx/1 -> MATLAB Function1/3(vx)
  [B] -> MATLAB Function1/8(B)
  [L2] -> MATLAB Function1/7(L2)
  Demux2/2 -> MATLAB Function1/2(delta2)
  wr/1 -> MATLAB Function1/5(wr)
  delta/1 -> Demux2/1
  [L1] -> MATLAB Function1/6(L1)
  Mux/1 -> vw/1
  MATLAB Function1/1(vw11) -> Mux/1
  MATLAB Function1/2(vw12) -> Mux/2
  MATLAB Function1/3(vw21) -> Mux/3
  MATLAB Function1/4(vw22) -> Mux/4

== matlab function model/vehicle/State observer/lamda/MATLAB Function2 ==
  data: vw input size=4; ww input size=4; s1 output; R input; s2 output; s3 output; s4 output
function [s1,s2,s3,s4] = fcn(vw,ww,R) 

s1 = (ww(1)*R-vw(1))/max(vw(1),ww(1)*R)*100;
s2 = (ww(2)*R-vw(2))/max(vw(2),ww(2)*R)*100;
s3 = (ww(3)*R-vw(3))/max(vw(3),ww(3)*R)*100;
s4 = (ww(4)*R-vw(4))/max(vw(4),ww(4)*R)*100;

== matlab function model/vehicle/tire/MATLAB Function3 ==
  data: alpha input size=4; s input size=4; Fz input size=4; Fx1 output; Fx2 output; Fx3 output; Fx4 output; Fy1 output; Fy2 output; Fy3 output; Fy4 output
function [Fx1,Fx2,Fx3,Fx4,Fy1,Fy2,Fy3,Fy4]= fcn(alpha,s,Fz)
alpha=alpha*180/pi;
miu=1;
%%纵向力与侧向力计算
% Cx=20000;
% Cy=30000;
% l11=miu*Fz(1)*(1+s(1))/2/sqrt((Cx*s(1))^2+(Cy*tan(alpha(1)))^2);
% l12=miu*Fz(2)*(1+s(2))/2/sqrt((Cx*s(2))^2+(Cy*tan(alpha(2)))^2);
% l21=miu*Fz(3)*(1+s(3))/2/sqrt((Cx*s(3))^2+(Cy*tan(alpha(3)))^2);
% l22=miu*Fz(4)*(1+s(4))/2/sqrt((Cx*s(4))^2+(Cy*tan(alpha(4)))^2);
% %状态函数判断
% if l11<1
%     f11=l11*(2-l11);
% else
%     f11=1;
% end
% if l12<1
%     f12=l12*(2-l12);
% else
%     f12=1;
% end
% if l21<1
%     f21=l21*(2-l21);
% else
%     f21=1;
% end
% if l22<1
%     f22=l22*(2-l22);
% else
%     f22=1;
% end
% %纵向力与横向力计算
% Fx1=Cx*s(1)*f11/(1+s(1));
% Fy1=Cy*tan(alpha(1))*f11/(1+s(1));
% Fx2=Cx*s(2)*f12/(1+s(2));
% Fy2=Cy*tan(alpha(2))*f12/(1+s(2));
% Fx3=Cx*s(3)*f21/(1+s(3));
% Fy3=Cy*tan(alpha(3))*f21/(1+s(3));
% Fx4=Cx*s(4)*f22/(1+s(4));
% Fy4=Cy*tan(alpha(4))*f22/(1+s(4));
Fz=Fz/1000;

%% 11
a1=-21.3;a2=1144;a3=49.6;a4=226;a5=0.069;a6=-0.006;a7=0.056;a8=0.486;
C=1.65;
D=a1*Fz(1)^2+a2*Fz(1);
BCD=(a3*Fz(1)^2+a4*Fz(1))/exp(a5*Fz(1));
B=BCD/(C*D);
E=a6*Fz(1)^2+a7*Fz(1)+a8;
Fx0=D*sin(C*atan(B*s(1)-E*(B*s(1)-atan(B*s(1)))));

a1=-22.1;a2=1011;a3=1078;a4=1.82;a5=0.208;a6=0;a7=-0.354;a8=0.707;
C1=1.3;
D1=a1*Fz(1)^2+a2*Fz(1);
BCD=a3.*sin(a4*atan(a5*Fz(1)));
B1=BCD/(C1*D1);
E1=a6*Fz(1)^2+a7*Fz(1)+a8;
Fy0=-D1*sin(C1*atan(B1*alpha(1)-E1*(B1*alpha(1)-atan(B1*alpha(1)))));

dx=s(1)/(100+abs(s(1)));
dy=100*tan(alpha(1)*pi/180)/(100+abs(s(1)));
d=sqrt(dx^2+dy^2);
Fx1=sign(s(1))*Fx0*dx/d;
% Fx1=Fx0*dx/d;
Fy1=sign(alpha(1))*Fy0*dy/d;

%% 12
a1=-21.3;a2=1144;a3=49.6;a4=226;a5=0.069;a6=-0.006;a7=0.056;a8=0.486;
C=1.65;
D=a1*Fz(2)^2+a2*Fz(2);
BCD=(a3*Fz(2)^2+a4*Fz(2))/exp(a5*Fz(2));
B=BCD/(C*D);
E=a6*Fz(2)^2+a7*Fz(2)+a8;
Fx0=D*sin(C*atan(B*s(2)-E*(B*s(2)-atan(B*s(2)))));

a1=-22.1;a2=1011;a3=1078;a4=1.82;a5=0.208;a6=0;a7=-0.354;a8=0.707;
C1=1.3;
D1=a1*Fz(2)^2+a2*Fz(2);
BCD=a3.*sin(a4*atan(a5*Fz(2)));
B1=BCD/(C1*D1);
E1=a6*Fz(2)^2+a7*Fz(2)+a8;
Fy0=-D1*sin(C1*atan(B1*alpha(2)-E1*(B1*alpha(2)-atan(B1*alpha(2)))));

dx=s(2)/(100+abs(s(2)));
dy=100*tan(alpha(2)*pi/180)/(100+abs(s(2)));
d=sqrt(dx^2+dy^2);
Fx2=sign(s(2))*Fx0*dx/d;
% Fx2=Fx0*dx/d;
Fy2=sign(alpha(2))*Fy0*dy/d;

%% 21
a1=-21.3;a2=1144;a3=49.6;a4=226;a5=0.069;a6=-0.006;a7=0.056;a8=0.486;
C=1.65;
D=a1*Fz(3)^2+a2*Fz(3);
BCD=(a3*Fz(3)^2+a4*Fz(3))/exp(a5*Fz(3));
B=BCD/(C*D);
E=a6*Fz(3)^2+a7*Fz(3)+a8;
Fx0=D*sin(C*atan(B*s(3)-E*(B*s(3)-atan(B*s(3)))));

a1=-22.1;a2=1011;a3=1078;a4=1.82;a5=0.208;a6=0;a7=-0.354;a8=0.707;
C1=1.3;
D1=a1*Fz(3)^2+a2*Fz(3);
BCD=a3.*sin(a4*atan(a5*Fz(3)));
B1=BCD/(C1*D1);
E1=a6*Fz(3)^2+a7*Fz(3)+a8;
Fy0=-D1*sin(C1*atan(B1*alpha(3)-E1*(B1*alpha(3)-atan(B1*alpha(3)))));

dx=s(3)/(100+abs(s(3)));
dy=100*tan(alpha(3)*pi/180)/(100+abs(s(3)));
d=sqrt(dx^2+dy^2);
Fx3=sign(s(3))*Fx0*dx/d;
% Fx3=Fx0*dx/d;
Fy3=sign(alpha(3))*Fy0*dy/d;

%% 22
a1=-21.3;a2=1144;a3=49.6;a4=226;a5=0.069;a6=-0.006;a7=0.056;a8=0.486;
C=1.65;
D=a1*Fz(4)^2+a2*Fz(4);
BCD=(a3*Fz(4)^2+a4*Fz(4))/exp(a5*Fz(4));
B=BCD/(C*D);
E=a6*Fz(4)^2+a7*Fz(4)+a8;
Fx0=D*sin(C*atan(B*s(4)-E*(B*s(4)-atan(B*s(4)))));

a1=-22.1;a2=1011;a3=1078;a4=1.82;a5=0.208;a6=0;a7=-0.354;a8=0.707;
C1=1.3;
D1=a1*Fz(4)^2+a2*Fz(4);
BCD=a3.*sin(a4*atan(a5*Fz(4)));
B1=BCD/(C1*D1);
E1=a6*Fz(4)^2+a7*Fz(4)+a8;
Fy0=-D1*sin(C1*atan(B1*alpha(4)-E1*(B1*alpha(4)-atan(B1*alpha(4)))));

dx=s(4)/(100+abs(s(4)));
dy=100*tan(alpha(4)*pi/180)/(100+abs(s(4)));
d=sqrt(dx^2+dy^2);
Fx4=sign(s(4))*Fx0*dx/d;
% Fx4=Fx0*dx/d;
Fy4=sign(alpha(4))*Fy0*dy/d;

== matlab function model/controler/Subsystem/MATLAB Function ==
  data: u1 input; f output; u2 input; r output
function [f,r] = fcn(u1,u2)
reald1=(u1-50)/100*284;
reald2=(u2-50)/100*284;
realf=reald1/6;
realr=reald2/6;
f=realf*pi/180;
r=realr*pi/180;

== matlab function model/driver/T_control/Acc_control ==
  data: u input; y output; v input
function y = fcn(u,v)
y=0;
if u>=2&&v>5
    y=0;
end
if u>=2&&v<=5
    y=u;
end
if u<2&&v>5
    y=0;
end
if u<2&&v<=5
    y=u;
end

== matlab function model/controler/Subsystem/Subsystem/MATLAB Function ==
  data: u1 input; y output; unused input
function y = fcn(u1,~)

y = (u1-50)/100*284;

== matlab function model/controler/Subsystem/Subsystem/MATLAB Function1 ==
  data: Td input; T output; ww input; p output
function [T,p] = fcn(Td,ww)
P0=Td(1)*ww(1)+Td(2)*ww(2)+Td(3)*ww(3)+Td(4)*ww(4);
if P0<=80000
    T=Td;
    p=P0;
else
    T=Td*80000/P0;
    p=T(1)*ww(1)+T(2)*ww(2)+T(3)*ww(3)+T(4)*ww(4);
end

== matlab function model/vehicle/State observer/wheel/MATLAB Function ==
  data: Td input size=4; ww1 output; Fx input size=4; Fz input size=4; Iw input; R input; f input; ww2 output; ww3 output; ww4 output
function [ww1,ww2,ww3,ww4]=fcn(Td,Fx,Fz,Iw,R,f)
ww1=(Td(1)-Fx(1)*R-Fz(1)*f*R)/Iw;
ww2=(Td(2)-Fx(2)*R-Fz(2)*f*R)/Iw;
ww3=(Td(3)-Fx(3)*R-Fz(3)*f*R)/Iw;
ww4=(Td(4)-Fx(4)*R-Fz(4)*f*R)/Iw;

== matlab function model/controler/Subsystem/Subsystem/MATLAB Function3 ==
  data: L1 input; e output; L2 input; m input; vx input; wreal input; delta1 input
function e = fcn(L1,L2,m,vx,wreal,delta1)
L=L1+L2;
k1=30000;
k2=30000;
K=m*(L1/k2-L2/k1)/L/L;
wref=vx*delta1*pi/180/L/(1+K*vx*vx)/6;
e=wref-wreal;

== matlab function model/driver/T_control/Tlimit ==
  data: basic input; y output; add input; soc input; J input
function y = fcn(basic,add,soc,J)
if soc<20&&J<30
    y=basic;
else
    y=basic+add;
end

== matlab function model/controler/Subsystem/Subsystem/二阶分配横向力矩 ==
  data: Td input; Fz input; Td1 output double size=1; Td2 output double size=1; Td3 output double size=1; Td4 output double size=1; tempL input; tempR input; M input; alpha input
function [Td1,Td2,Td3,Td4]  = fcn(Td,Fz,tempL,tempR,M,alpha)
l1=1.23;
l2=1.2;
temp=max(tempL,tempR);
FZ=Fz(1)+Fz(2)+Fz(3)+Fz(4);
if abs(alpha)<10
    if temp<=40
        Td1=Fz(1)/(FZ)*Td;
        Td2=Fz(2)/(FZ)*Td;
        Td3=Fz(3)/(FZ)*Td;
        Td4=Fz(4)/(FZ)*Td;
    else
        Td1=Fz(1)/(FZ)*Td*40/temp;
        Td2=Fz(2)/(FZ)*Td*40/temp;
        Td3=Fz(3)/(FZ)*Td*40/temp;
        Td4=Fz(4)/(FZ)*Td*40/temp;
    end
else
    if temp<=40
        Td1=Fz(1)/(FZ)*Td+M/(2*l1*cos(alpha*pi/284));
        Td2=Fz(2)/(FZ)*Td-M/(2*l1*cos(alpha*pi/284));
        Td3=Fz(3)/(FZ)*Td+M/(2*l2);
        Td4=Fz(4)/(FZ)*Td-M/(2*l2);
    else
        Td1=(Fz(1)/(FZ)*Td+M/(2*l1*cos(alpha*pi/284)))*40/temp;
        Td2=(Fz(2)/(FZ)*Td-M/(2*l1*cos(alpha*pi/284)))*40/temp;
        Td3=(Fz(3)/(FZ)*Td+M/(2*l2))*40/temp;
        Td4=(Fz(4)/(FZ)*Td-M/(2*l2))*40/temp;
    end
end

== matlab function model/vehicle/vehicle_body/MATLAB Function2 ==
  data: vx input; Fx output; Fy output; Fx11 input; Mz output; Fx12 input; Fx21 input; Fx22 input; Fy11 input; Fy12 input; Fy21 input; Fy22 input; delta1 input; delta2 input; L1 input; L2 input; B input
function [Fx,Fy,Mz] = fcn(vx,Fx11,Fx12,Fx21,Fx22,Fy11,Fy12,Fy21,Fy22,delta1,delta2,L1,L2,B)
Fx=(Fx11+Fx12)*cos(delta1)+(Fx21+Fx22)*cos(delta2)-(Fy11+Fy12)*sin(delta1)-(Fy21+Fy22)*sin(delta2)-0.5*1.6*1.2*1.162*vx*vx;
%%侧向控制
Fy=(Fx11+Fx12)*sin(delta1)+(Fx21+Fx22)*sin(delta2)+(Fy11+Fy12)*cos(delta1)+(Fy21+Fy22)*cos(delta2);
%%横摆控制
Mz=Fx11*sin(delta1)*L1- Fx11*cos(delta1)*B/2+Fy11*sin(delta1)*B/2+Fy11*cos(delta1)*L1...
     +Fx12*sin(delta1)*L1+Fx12*cos(delta1)*B/2- Fy12*sin(delta1)*B/2+Fy12*cos(delta1)*L1...
     - Fx21*sin(delta2)*L2-Fx21*cos(delta2)*B/2+Fy21*sin(delta2)*B/2- Fy21*cos(delta2)*L2...
     - Fx22*sin(delta2)*L2+Fx22*cos(delta2)*B/2- Fy22*sin(delta2)*B/2- Fy22*cos(delta2)*L2;

== matlab function model/vehicle/State observer/alpha&vw/lunsu/MATLAB Function1 ==
  data: delta1 input; vw11 output size=1; delta2 input; vx input; vy input; wr input; L1 input; vw12 output size=1; vw21 output size=1; vw22 output size=1; L2 input; B input
function [vw11,vw12,vw21,vw22] = wheelspeed(delta1,delta2,vx,vy,wr,L1,L2,B)
vw11 = ((vx-(B/2)*wr)*cos(delta1)+(vy+L1*wr)*sin(delta1));
vw12 = ((vx+(B/2)*wr)*cos(delta1)+(vy+L1*wr)*sin(delta1));
vw21 = ((vx-(B/2)*wr)*cos(delta2)+(vy-L2*wr)*sin(delta2));
vw22 = ((vx+(B/2)*wr)*cos(delta2)+(vy-L2*wr)*sin(delta2));

== matlab function model/vehicle/State observer/alpha&vw/cepianjiao/MATLAB Function ==
  data: delta1 input; alpha1 output size=1; delta2 input; vx input; vy input; wr input; L1 input; L2 input; alpha2 output size=1; alpha3 output size=1; alpha4 output size=1; B input
function [alpha1,alpha2,alpha3,alpha4] = fcn(delta1,delta2,vx,vy,wr,L1,L2,B)
alpha1 = atan((vy+L1*wr)/(vx-(B/2)*wr))-delta1;
alpha2 = atan((vy+L1*wr)/(vx+(B/2)*wr))-delta1;
alpha3 = atan((vy-L2*wr)/(vx-(B/2)*wr))-delta2;
alpha4 = atan((vy-L2*wr)/(vx+(B/2)*wr))-delta2;

== matlab function model/vehicle/State observer/Fz/fun2 MATLAB Function ==
  data: ax input; ay input; vx input; m input; g input; B input; h input; Fz11 output size=1; Fz12 output size=1; Fz21 output size=1; L1 input; L2 input; Fz22 output size=1; FW input; RW input
function [Fz11,Fz12,Fz21,Fz22]= fcn(ax,ay,vx,m,g,B,h,L1,L2,FW,RW)
FA=2.07*vx*vx*0.5*1.162;
RA=2.07*vx*vx*0.7*1.162;
Fz1=(L2*(g*m+FA+RA)+FA*FW-RA*RW-ax*h*m)/(L1 + L2);
Fz2=(L1*(g*m+FA+RA)-FA*FW+RA*RW+ax*h*m)/(L1 + L2);
Fz11=(Fz1*(B*g-2*ay*h))/(2*B*g);
Fz12=(Fz1*(B*g+2*ay*h))/(2*B*g);
Fz21=(Fz2*(B*g-2*ay*h))/(2*B*g);
Fz22=(Fz2*(B*g+2*ay*h))/(2*B*g);
